simulink model "DSBAModulator"  (R2020b)
settings: Solver=FixedStepAuto  StartTime=0.0  StopTime=0.1  RelTol=1e-3
settings Model: PacingRate=0.011000  Creator=DAM  LastModifiedBy=DAM

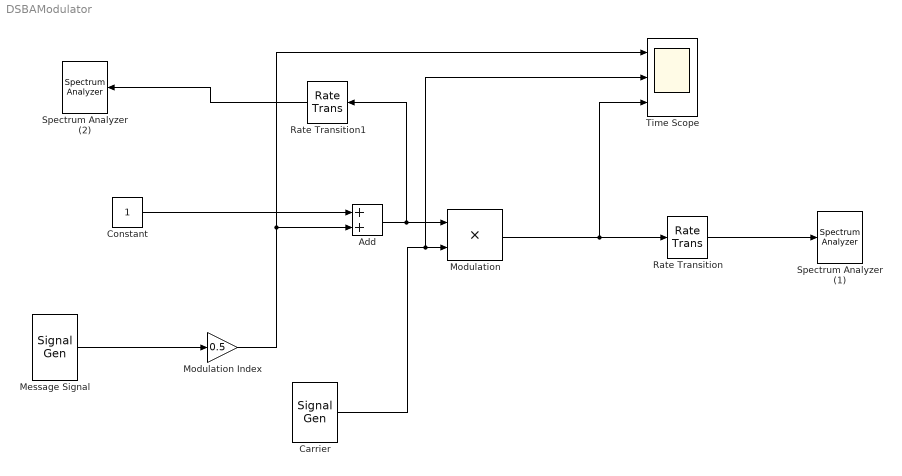
== system DSBAModulator ==
  Add : Sum
  Carrier : SignalGenerator  Frequency=20000
  Constant : Constant
  Message Signal : SignalGenerator  Frequency=1000
  Modulation : Product
  "Modulation Index " : Gain  Gain=0.5
  Rate Transition : RateTransition
  Rate Transition1 : RateTransition
  Spectrum Analyzer (1) : SpectrumAnalyzer
  Spectrum Analyzer (2) : SpectrumAnalyzer
  Time Scope : Scope  NumInputPorts=3
  wires:
  Add/1 -> Modulation/1, Rate Transition1/1
  Rate Transition1/1 -> Spectrum Analyzer (2)/1
  "Modulation Index "/1 -> Time Scope/1, Add/2
  Constant/1 -> Add/1
  Message Signal/1 -> "Modulation Index "/1
  Carrier/1 -> Time Scope/2, Modulation/2
  Modulation/1 -> Time Scope/3, Rate Transition/1
  Rate Transition/1 -> Spectrum Analyzer (1)/1
